simulink model "CML_Dyanmic_Sensory_Weighting"  (R2015a)
settings: Solver=ode4  SolverMode=MultiTasking  StartTime=0.0  StopTime=inf  FixedStep=BKIN_STEP_TIME  RelTol=1e-3
StartFcn:
  |  warndlg('Dexterit-E models cannot run under simulation. Please compile your model and run it from within Dexterit-E.');set_param(bdroot,'SimulationCommand','stop')
model workspace (MAT data in the model file):
  col_x = 1
  col_y = 2
  RADIUS_VIS = 3
  COLOR_INIT = 4
  START_TARGET_COL = 1
  DELAY_POST_TRIAL_COL = 17
  BKIN_STEP_TIME = 0.00025
  COLOR_MOVE = 5
  START_WAIT_TIME_COL = 2
  STIM_DUR_COL = 13
  MAX_MOVE_TIME_COL = 14
  HOLD_TIME_COL = 15
  E_START_TRIAL = 2
  E_START_REACHED = 4
  E_MOVED_EARLY = 21
  E_GO_CUE = 9
  E_MOVE_TIMEOUT = 23
  E_HOLDING_STILL = 12
  E_END_TRIAL = 14
  CONTROL_PT3_COL = 10
  STROKE_WIDTH = 6
  K_HAND_VEL = 1
  E_MOVE_ON = 10
  CUE_TYPE_COL = 6
  HAND_VIS_COL = 5
  K_HOLDTIME = 2
  K_ROBOT_RAMP_TIME = 3
  E_ROBOT_RETURN_TO_START = 33
  E_ENABLED_CONTROLLER = 31
  K_TIME_TO_START = 4
  E_RETURN_TO_START = 35
  E_HOLD_POS = 37
  E_INCREMENTING_TSTEP1 = 6
  E_INCREMENTING_TSTEP2 = 7
  E_INCREMENTING_TSTEP3 = 8
  CONTROL_PT0_COL = 7
  BKIN_KINEMATIC_FRAME_SIZE = 400
  E_NO_EVENT = 0
  E_BUTTON_ON = 40
  CONTROL_PTV1_COL = 8
  CONTROL_PTV2_COL = 9
  CONTROL_PTP1_COL = 11
  CONTROL_PTP2_COL = 12
  REACH_TARGET_COL = 3
  VIS_TARGET_COL = 4
  RADIUS_LOGICAL = 7
  FEEDBACK_TIME_COL = 16
  K_HAND_TARGET = 5
  E_SHOW_FEEDBACK = 16
  K_MIDPOINTY = 6
  K_MIDPOINT_Y = 6
  K_ARC_FDBK_TARGET = 7
  TEXT1 = 8
  TEXT2 = 9
  TEXT3 = 10
  K_CUE_TARGET = 8
  CONTINUE = 4
  TEXT4 = 11
  E_PAUSE = 41
libraries: slrtlib x10, Video x9, General x3, KINARM_general x3, KINARM_loads x2, xpcnilib x1
(part 1 of 2)
CloseFcn:
  | rtwprivate ssgencode ModelCloseRequest b2lab2d
settings Model: xpc_rtwmakecfg_data=_xpcethercatlib_  ModifiedComment=chris -- Wed Feb 16 09:18:30 2005 -- Version 1.1384  ModifiedHistory=Feb 16/05 - Add error repeat, add offset ramp  ExtModeArmWhenConnect=off  ExtModeLogAll=off  Creator=Chris Grebeldinger  LastModifiedBy=User
settings SolverCC: EnableConcurrentExecution=on  AutoInsertRateTranBlk=on
settings DataIOCC: LimitDataPoints=off  SignalLoggingSaveFormat=ModelDataLogs  SaveOutput=off  SaveTime=off  SignalLoggingName=sigsOut
settings OptimizationCC: BlockReduction=off  BooleanDataType=off  OptimizeBlockIOStorage=off  BufferReuse=off  GlobalBufferReuse=off  ExpressionFolding=off  ExpressionDepthLimit=2147483647  LocalBlockOutputs=off  InitFltsAndDblsToZero=on
settings DebuggingCC: SaveWithParameterizedLinksMsg=none  UnderspecifiedInitializationDetection=Classic  MergeDetectMultiDrivingBlocksExec=none  SignalResolutionControl=TryResolveAllWithWarning  MultiTaskDSMMsg=warning  FcnCallInpInsideContextMsg=UseLocalSettings  StateNameClashWarn=warning  StrictBusMsg=ErrorOnBusTreatedAsVector
settings HardwareCC: ProdIntDivRoundTo=Zero  ProdEndianess=LittleEndian  ProdLongLongMode=on  ProdHWDeviceType=Generic->32-bit x86 compatible  TargetHWDeviceType=32-bit Generic
settings SFSimCC: SimCustomHeaderCode="#include \"stdlib.h\""  SFSimEcho=off  SimParseCustomCode=off
settings RTWCC: SystemTargetFile=slrt.tlc  TemplateMakefile=slrt_default_tmf  Description=Simulink Real-Time  CustomSourceCode="#include \"stdlib.h\""
settings CodeAppCC: MaxIdLength=63
settings SimulinkRealTimeCC: TargetFcnLib=ansi_tfl_tmw.mat  GeneratePreprocessorConditionals=Disable all  xPCisDownloadable=off  xPCisDefaultEnv=off

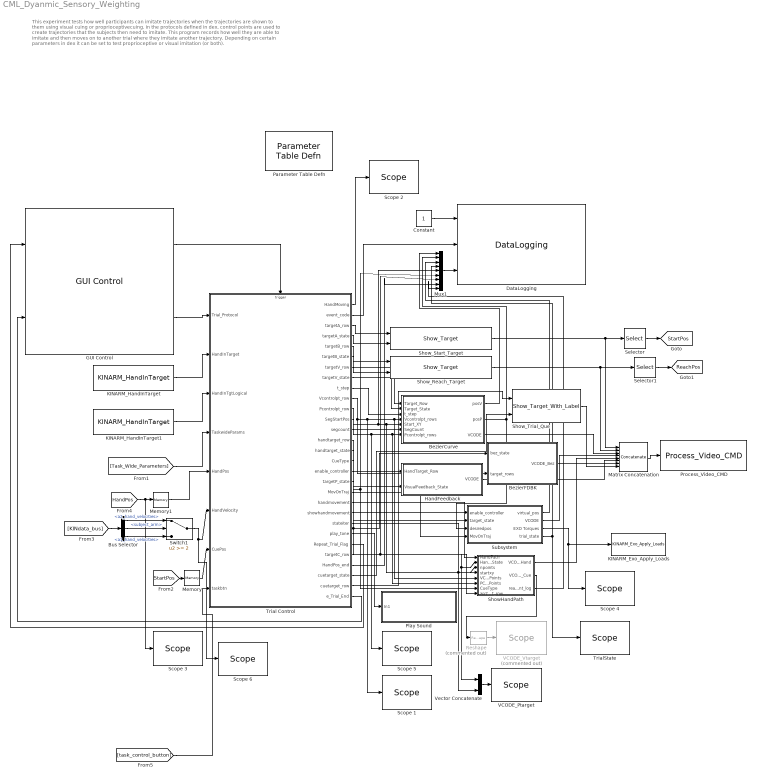
== system CML_Dyanmic_Sensory_Weighting ==
  note: This experiment tests how well participants can imitate trajectories when the trajectories
      | are shown to them using visual cuing or proprioceptivecuing. In the protocols defined in
      | dex, control points are used to create trajectories that the subjects then need to imitate.
      | This program records how well they are able to imitate and then moves on to another trial
      | where they imitate another trajectory. Depending on certain parameters in dex it can be
      | set to test proprioceptive or visual imitation (or both).
  BezierCurve : Subsystem
  BezierFDBK : Subsystem
  Bus Selector : BusSelector  OutputSignals=Robot2.a2_hand_velocities,KINDataGeneral.subject_arm,Robot1.a1_hand_velocities
  Constant : Constant
  DataLogging : General/DataLogging  log_event_codes=on  log_analog_inputs=on  show_time_remaining=off  ecat_include=on
  GUI Control : General/GUI Control  task_version=1.0  show_repeat_trial_flag=on  use_custom_tp=off  target_type_str=Circle  Target_Type=1  XYcols=[1 2]  Vcols=3  Lcols=4  indices_padding=[0 0 0 0;0 0 0 0]  target_table_rows=64  load_table_rows=20  tp_table_rows=100
  HandFeedback : Subsystem
  KINARM_Exo_Apply_Loads : KINARM_loads/KINARM_Exo_Apply_Loads  up_duration=200  down_duration=200  max_torque=5  limit_motors=off
  KINARM_HandInTarget : KINARM_general/KINARM_HandInTarget  use_dominant_hand=on  target_type=Circle  num_states=1  attribcol1=[RADIUS_VIS]  attribcol2=[0]  attribcol3=[0]  attribcol4=[0]  attribcol5=[0]
  KINARM_HandInTarget1 : KINARM_general/KINARM_HandInTarget  use_dominant_hand=on  target_type=Circle  num_states=1  attribcol1=[RADIUS_LOGICAL]  attribcol2=[0]  attribcol3=[0]  attribcol4=[0]  attribcol5=[0]
  Matrix Concatenation : Concatenate  NumInputs=8  Mode=Multidimensional array
  Memory : Memory
  Memory1 : Memory
  Mux1 : Mux  Inputs=9
  Parameter Table Defn : General/Parameter Table Defn  ShowInLibBrowser=0
  Play Sound : Subsystem
  Process_Video_CMD : Video/Process_Video_CMD  video_delay=50
  Reshape : Reshape  Commented=on
  Scope 1 : slrtlib/Displays and Logging/Scope   scopeno=7  scopetype=Target  autostart=on  viewmode=Numerical  formatstr='%15.6f'  grid=on  ylimits=[0,0]  nosamples=250  noprepostsamples=0  interleave=1  triggermode=FreeRun  triggersignal=1  trigsignalfromport=off  triggerlevel=0.0  triggerslope=Either  triggerscope=1  triggersample=0  filename=data.dat  mode=Lazy  writesize=512  autorestart=off  dynamicfilemode=off  maxwritefilesize=512*1024^2
  Scope 2 : slrtlib/Displays and Logging/Scope   scopeno=2  scopetype=Target  autostart=on  viewmode=Numerical  formatstr='%15.6f'  grid=on  ylimits=[0,0]  nosamples=250  noprepostsamples=0  interleave=1  triggermode=FreeRun  triggersignal=1  trigsignalfromport=off  triggerlevel=0.0  triggerslope=Either  triggerscope=1  triggersample=0  filename=data.dat  mode=Lazy  writesize=512  autorestart=off  dynamicfilemode=off  maxwritefilesize=512*1024^2
  Scope 3 : slrtlib/Displays and Logging/Scope   scopeno=3  scopetype=Target  autostart=on  viewmode=Numerical  formatstr='%15.6f'  grid=on  ylimits=[0,0]  nosamples=250  noprepostsamples=0  interleave=1  triggermode=FreeRun  triggersignal=1  trigsignalfromport=off  triggerlevel=0.0  triggerslope=Either  triggerscope=1  triggersample=0  filename=data.dat  mode=Lazy  writesize=512  autorestart=off  dynamicfilemode=off  maxwritefilesize=512*1024^2
  Scope 4 : slrtlib/Displays and Logging/Scope   scopeno=6  scopetype=Target  autostart=on  viewmode=Numerical  formatstr='%15.6f'  grid=on  ylimits=[0,0]  nosamples=250  noprepostsamples=0  interleave=1  triggermode=FreeRun  triggersignal=1  trigsignalfromport=off  triggerlevel=0.0  triggerslope=Either  triggerscope=1  triggersample=0  filename=data.dat  mode=Lazy  writesize=512  autorestart=off  dynamicfilemode=off  maxwritefilesize=512*1024^2
  Scope 5 : slrtlib/Displays and Logging/Scope   scopeno=8  scopetype=Target  autostart=on  viewmode=Numerical  formatstr='%15.6f'  grid=on  ylimits=[0,0]  nosamples=250  noprepostsamples=0  interleave=1  triggermode=FreeRun  triggersignal=1  trigsignalfromport=off  triggerlevel=0.0  triggerslope=Either  triggerscope=1  triggersample=0  filename=data.dat  mode=Lazy  writesize=512  autorestart=off  dynamicfilemode=off  maxwritefilesize=512*1024^2
  Scope 6 : slrtlib/Displays and Logging/Scope   scopeno=4  scopetype=Target  autostart=on  viewmode=Numerical  formatstr='%15.6f'  grid=on  ylimits=[0,0]  nosamples=250  noprepostsamples=0  interleave=1  triggermode=FreeRun  triggersignal=1  trigsignalfromport=off  triggerlevel=0.0  triggerslope=Either  triggerscope=1  triggersample=0  filename=data.dat  mode=Lazy  writesize=512  autorestart=off  dynamicfilemode=off  maxwritefilesize=512*1024^2
  Selector : Selector  InputPortWidth=70  Indices=[3 4]
  Selector1 : Selector  InputPortWidth=70  Indices=[3 4]
  ShowHandPath : Subsystem
  Show_Reach_Target : Video/Show_Target  target_type=Rectangle  num_states=1  attribcol1=[0 COLOR_INIT STROKE_WIDTH RADIUS_VIS RADIUS_VIS 0]  attribcol2=[0 0 0 0 0 0]  attribcol3=[0 0 0 0 0 0]  attribcol4=[0 0 0 0 0 0]  attribcol5=[0 0 0 0 0 0]  stateindices_padding=[0 0 0 0 0;0 0 0 0 0;0 0 0 0 0;0 0 0 0 0;0 0 0 0 0]  source=dialog  opacity=100  target_display=Both subject and operator displays  num_col=6
  Show_Start_Target : Video/Show_Target  target_type=Rectangle  num_states=1  attribcol1=[0 COLOR_INIT STROKE_WIDTH RADIUS_VIS RADIUS_VIS 0]  attribcol2=[0 0 0 0 0 0]  attribcol3=[0 0 0 0 0 0]  attribcol4=[0 0 0 0 0 0]  attribcol5=[0 0 0 0 0 0]  stateindices_padding=[0 0 0 0 0;0 0 0 0 0;0 0 0 0 0;0 0 0 0 0;0 0 0 0 0]  source=dialog  opacity=100  target_display=Both subject and operator displays  num_col=6
  Show_Trial_Que : Video/Show_Target_With_Label  target_type=Circle  num_states=4  attribcol1=[0 0 0 RADIUS_VIS TEXT1 COLOR_INIT STROKE_WIDTH]  attribcol2=[0 0 0 RADIUS_VIS TEXT2 COLOR_INIT STROKE_WIDTH]  attribcol3=[0 0 0 RADIUS_VIS TEXT3 COLOR_INIT STROKE_WIDTH]  attribcol4=[0 0 0 RADIUS_VIS TEXT4 COLOR_INIT STROKE_WIDTH]  attribcol5=[0 0 0 0 0 0 0]  stateindices_padding=[0 0 0 0;0 0 0 0;0 0 0 0;0 0 0 0;0 0 0 0]  source=dialog  opacity=100  target_display=Both subject and operator displays
  Subsystem : Subsystem
  Switch1 : Switch  Threshold=2
  Trial Control : Stateflow chart  TreatAsAtomicUnit=on
  TrialState : slrtlib/Displays and Logging/Scope   scopeno=1  scopetype=Target  autostart=on  viewmode=Numerical  formatstr='%15.6f'  grid=on  ylimits=[0,0]  nosamples=250  noprepostsamples=0  interleave=1  triggermode=FreeRun  triggersignal=1  trigsignalfromport=off  triggerlevel=0.0  triggerslope=Either  triggerscope=1  triggersample=0  filename=data.dat  mode=Lazy  writesize=512  autorestart=off  dynamicfilemode=off  maxwritefilesize=512*1024^2
  VCODE_Ptarget : slrtlib/Displays and Logging/Scope   scopeno=5  scopetype=Target  autostart=on  viewmode=Numerical  formatstr='%15.6f'  grid=on  ylimits=[0,0]  nosamples=250  noprepostsamples=0  interleave=1  triggermode=FreeRun  triggersignal=1  trigsignalfromport=off  triggerlevel=0.0  triggerslope=Either  triggerscope=1  triggersample=0  filename=data.dat  mode=Lazy  writesize=512  autorestart=off  dynamicfilemode=off  maxwritefilesize=512*1024^2
  VCODE_Vtarget : slrtlib/Displays and Logging/Scope   Commented=on  scopeno=4  scopetype=Target  autostart=on  viewmode=Numerical  formatstr='%15.6f'  grid=on  ylimits=[0,0]  nosamples=250  noprepostsamples=0  interleave=1  triggermode=FreeRun  triggersignal=1  trigsignalfromport=off  triggerlevel=0.0  triggerslope=Either  triggerscope=1  triggersample=0  filename=data.dat  mode=Lazy  writesize=512  autorestart=off  dynamicfilemode=off  maxwritefilesize=512*1024^2
  Vector Concatenate : Concatenate
  tag scope: ReachPos=global, StartPos=global
  wires:
  Trial Control/29(e_Trial_End) -> GUI Control/2
  Trial Control/4(targetA_state) -> Show_Start_Target/2
  Trial Control/3(targetA_row) -> Show_Start_Target/1
  Matrix Concatenation/1 -> Process_Video_CMD/1
  Trial Control/2(event_code) -> DataLogging/2
  Constant/1 -> DataLogging/1
  GUI Control/2 -> Trial Control/1(Trial_Protocol)
  KINARM_HandInTarget/1 -> Trial Control/2(HandInTarget)
  Trial Control/14(handtarget_row) -> HandFeedback/1(HandTarget_Row)
  Trial Control/15(handtarget_state) -> HandFeedback/2(VisualFeedback_State)
  Show_Start_Target/1 -> Matrix Concatenation/1, Selector/1
  Trial Control/24(Repeat_Trial_Flag) -> GUI Control/1
  [Task_Wide_Parameters] -> Trial Control/4(TaskwideParams)
  Trial Control/9(t_step) -> BezierCurve/3(t_step)
  Trial Control/7(targetV_row) -> BezierCurve/1(Target_Row)
  Trial Control/10(Vcontrolpt_row) -> BezierFDBK/2(target_rows), ShowHandPath/5(VControl_Points), BezierCurve/4(Vcontrolpt_rows), Scope 1/1
  Trial Control/1(HandMoving) -> Scope 2/1
  Switch1/1 -> Scope 6/1, Trial Control/6(HandVelocity)
  Trial Control/17(enable_controller) -> Subsystem/1(enable_controller)
  Trial Control/19(MovOnTraj) -> Subsystem/4(MovOnTraj)
  Mux1/1 -> DataLogging/3
  Subsystem/1(virtual_pos) -> Mux1/3
  Subsystem/3(EXO Torques) -> Scope 4/1, KINARM_Exo_Apply_Loads/1
  Subsystem/2(VCODE) -> Matrix Concatenation/4
  BezierCurve/3(VCODE) -> Matrix Concatenation/3
  Subsystem/4(trial_state) -> TrialState/1, Mux1/4
  [KINdata_bus] -> Bus Selector/1
  Trial Control/8(targetV_state) -> BezierCurve/2(Target_State)
  Trial Control/12(SegStartPos) -> Mux1/5, ShowHandPath/4(startxy), BezierCurve/5(Start_XY)
  HandFeedback/1(VCODE) -> Matrix Concatenation/6
  BezierCurve/1(posV) -> Mux1/1
  Memory/1 -> Trial Control/7(CuePos)
  Trial Control/13(segcount) -> BezierCurve/6(SegCount)
  Trial Control/23(play_tone) -> Play Sound/1(In1)
  GUI Control/1 -> Trial Control/Trigger
  BezierCurve/2(posP) -> Mux1/2, Subsystem/3(desiredpos)
  Trial Control/18(targetP_state) -> Subsystem/2(target_state)
  Trial Control/11(Pcontrolpt_row) -> Scope 5/1, ShowHandPath/6(PControl_Points), BezierCurve/7(Pcontrolpt_rows)
  Selector/1 -> [StartPos]
  [StartPos] -> Memory/1
  Trial Control/5(targetB_row) -> Show_Reach_Target/1
  Trial Control/6(targetB_state) -> Show_Reach_Target/2
  KINARM_HandInTarget1/1 -> Trial Control/3(HandInTgtLogical)
  Trial Control/16(CueType) -> ShowHandPath/7(CueType), Mux1/6
  [HandPos] -> Scope 3/1, Memory1/1
  Memory1/1 -> Trial Control/5(HandPos)
  Trial Control/20(handmovement) -> ShowHandPath/1(HandPath)
  Trial Control/21(showhandmovement) -> BezierFDBK/1("bez_state "), Vector Concatenate/1, ShowHandPath/2(HandPathState), Mux1/7
  ShowHandPath/1(VCODE_Hand) -> Matrix Concatenation/5
  Trial Control/22(stateiter) -> Vector Concatenate/2, ShowHandPath/3(npoints)
  Vector Concatenate/1 -> VCODE_Ptarget/1
  Reshape/1 -> VCODE_Vtarget/1
  ShowHandPath/3("reachmidpoint_log ") -> Mux1/9
  Trial Control/25(targetC_row) -> ShowHandPath/8(arctarget_row)
  Show_Reach_Target/1 -> Selector1/1, Matrix Concatenation/2
  Selector1/1 -> [ReachPos]
  BezierFDBK/1(VCODE_Bez) -> Matrix Concatenation/7
  Bus Selector/3 -> Switch1/3  "<a1_hand_velocities>"
  Bus Selector/2 -> Switch1/2  "<subject_arm>"
  Bus Selector/1 -> Switch1/1  "<a2_hand_velocities>"
  Trial Control/26(HandPos_end) -> Mux1/8
  ShowHandPath/2(VCODE_Cue) -> Reshape/1
  Show_Trial_Que/1 -> Matrix Concatenation/8
  Trial Control/27(cuetarget_state) -> Show_Trial_Que/2
  Trial Control/28(cuetarget_row) -> Show_Trial_Que/1
  [task_control_button] -> Trial Control/8(taskbtn)

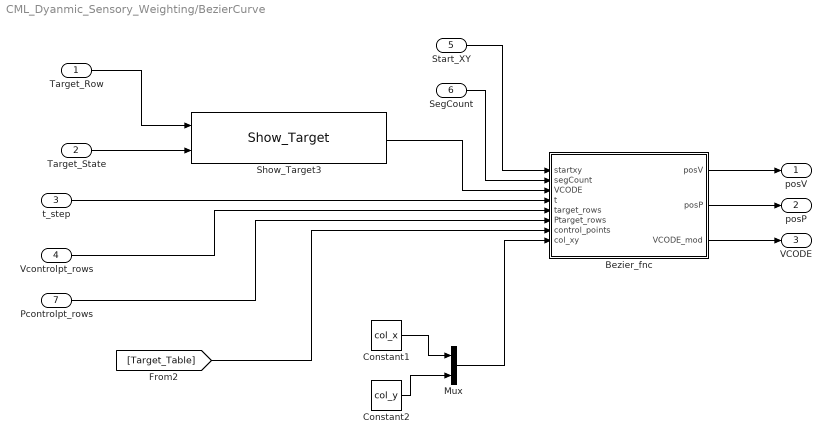
== system CML_Dyanmic_Sensory_Weighting/BezierCurve ==
  Target_Row : Inport
  Target_State : Inport  Port=2
  t_step : Inport  Port=3
  Vcontrolpt_rows : Inport  Port=4
  Start_XY : Inport  Port=5
  SegCount : Inport  Port=6
  Pcontrolpt_rows : Inport  Port=7
  Bezier_fnc : MATLAB Function  TreatAsAtomicUnit=on
  Constant1 : Constant  Value=col_x
  Constant2 : Constant  Value=col_y
  Mux : Mux  Inputs=2
  Show_Target3 : Video/Show_Target  target_type=Circle  num_states=1  attribcol1=[COLOR_INIT 0 0 RADIUS_VIS]  attribcol2=[0 0 0 0]  attribcol3=[0 0 0 0]  attribcol4=[0 0 0 0]  attribcol5=[0 0 0 0]  stateindices_padding=[0 0 0 0 0 0 0;0 0 0 0 0 0 0;0 0 0 0 0 0 0;0 0 0 0 0 0 0;0 0 0 0 0 0 0]  source=dialog  opacity=100  target_display=Both subject and operator displays  num_col=4
  posV : Outport
  posP : Outport  Port=2
  VCODE : Outport  Port=3
  wires:
  Show_Target3/1 -> Bezier_fnc/3(VCODE)
  Bezier_fnc/3(VCODE_mod) -> VCODE/1
  t_step/1 -> Bezier_fnc/4(t)
  [Target_Table] -> Bezier_fnc/7(control_points)
  Vcontrolpt_rows/1 -> Bezier_fnc/5(target_rows)
  Bezier_fnc/1(posV) -> posV/1
  Target_Row/1 -> Show_Target3/1
  Target_State/1 -> Show_Target3/2
  Mux/1 -> Bezier_fnc/8(col_xy)
  Constant1/1 -> Mux/1
  Constant2/1 -> Mux/2
  Start_XY/1 -> Bezier_fnc/1(startxy)
  SegCount/1 -> Bezier_fnc/2(segCount)
  Bezier_fnc/2(posP) -> posP/1
  Pcontrolpt_rows/1 -> Bezier_fnc/6(Ptarget_rows)

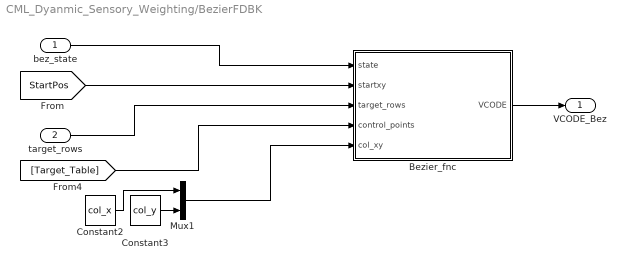
== system CML_Dyanmic_Sensory_Weighting/BezierFDBK ==
  "bez_state " : Inport
  target_rows : Inport  Port=2
  Bezier_fnc : MATLAB Function  TreatAsAtomicUnit=on
  Constant2 : Constant  Value=col_x
  Constant3 : Constant  Value=col_y
  Mux1 : Mux  Inputs=2
  VCODE_Bez : Outport
  wires:
  [Target_Table] -> Bezier_fnc/4(control_points)
  "bez_state "/1 -> Bezier_fnc/1(state)
  Constant2/1 -> Mux1/1
  Constant3/1 -> Mux1/2
  Mux1/1 -> Bezier_fnc/5(col_xy)
  target_rows/1 -> Bezier_fnc/3(target_rows)
  Bezier_fnc/1(VCODE) -> VCODE_Bez/1
  [StartPos] -> Bezier_fnc/2(startxy)

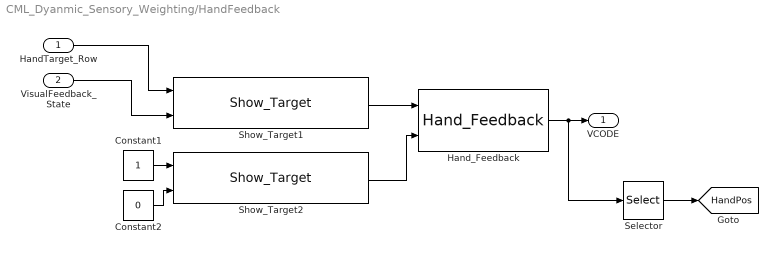
== system CML_Dyanmic_Sensory_Weighting/HandFeedback ==
  HandTarget_Row : Inport
  VisualFeedback_State : Inport  Port=2
  Constant1 : Constant
  Constant2 : Constant  Value=0
  Hand_Feedback : KINARM_general/Hand_Feedback  feedback_cntl_src=style and status
  Selector : Selector  NumberOfDimensions=2  InputPortWidth=70  IndexOptions=Index vector (dialog),Index vector (dialog)  Indices=1,[3 4]  OutputSizes=1,1
  Show_Target1 : Video/Show_Target  target_type=Circle  num_states=2  attribcol1=[COLOR_INIT 0 0 RADIUS_VIS]  attribcol2=[COLOR_MOVE 0 0 RADIUS_VIS]  attribcol3=[0 0 0 0]  attribcol4=[0 0 0 0]  attribcol5=[0 0 0 0]  stateindices_padding=[0 0 0 0 0 0 0;0 0 0 0 0 0 0;0 0 0 0 0 0 0;0 0 0 0 0 0 0;0 0 0 0 0 0 0]  source=dialog  opacity=100  target_display=Both subject and operator displays  num_col=4
  Show_Target2 : Video/Show_Target  target_type=Circle  num_states=2  attribcol1=[COLOR_INIT 0 0 RADIUS_VIS]  attribcol2=[COLOR_MOVE 0 0 RADIUS_VIS]  attribcol3=[0 0 0 0]  attribcol4=[0 0 0 0]  attribcol5=[0 0 0 0]  stateindices_padding=[0 0 0 0 0 0 0;0 0 0 0 0 0 0;0 0 0 0 0 0 0;0 0 0 0 0 0 0;0 0 0 0 0 0 0]  source=dialog  opacity=100  target_display=Both subject and operator displays  num_col=4
  VCODE : Outport
  tag scope: HandPos=global
  wires:
  Show_Target1/1 -> Hand_Feedback/1
  HandTarget_Row/1 -> Show_Target1/1
  VisualFeedback_State/1 -> Show_Target1/2
  Constant1/1 -> Show_Target2/1
  Constant2/1 -> Show_Target2/2
  Show_Target2/1 -> Hand_Feedback/2
  Hand_Feedback/1 -> Selector/1, VCODE/1
  Selector/1 -> [HandPos]

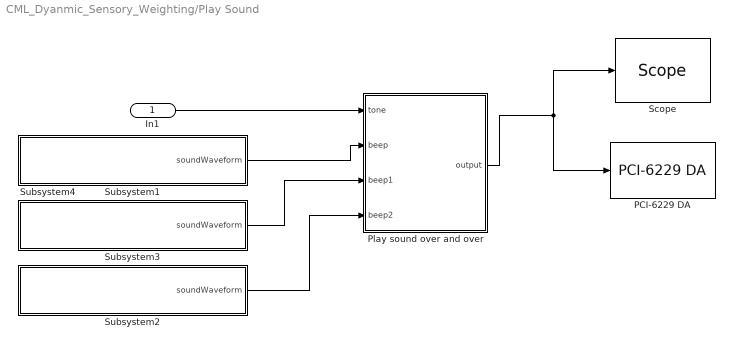
== system CML_Dyanmic_Sensory_Weighting/Play Sound ==
  In1 : Inport
  PCI-6229 DA : xpcnilib/D//A/M Series/PCI-6229 DA  channel=[1]  reset=[1]  initValue=[0]  sampletime=-1  slot=-1
  Play sound over and over : MATLAB Function  TreatAsAtomicUnit=on
  "Scope " : slrtlib/Displays and Logging/Scope   scopeno=9  scopetype=Target  autostart=on  viewmode=Graphical redraw  formatstr='%15.6f'  grid=on  ylimits=[0,0]  nosamples=4000  noprepostsamples=0  interleave=1  triggermode=FreeRun  triggersignal=1  trigsignalfromport=off  triggerlevel=0.0  triggerslope=Either  triggerscope=1  triggersample=0  filename=data.dat  mode=Lazy  writesize=512  autorestart=off  dynamicfilemode=off  maxwritefilesize=512*1024^2
  Subsystem1 : Subsystem  mask(Load Waveform Into Variable){fileName=beep}
      mask prompts: fileName "Name of .mat Data File (must be in current directory)"
      mask help: This block will load the .MAT file specified in the dialog, and put the first variable into a GoTo called 'soundWaveform'.
      mask init:
      | filenameFromMask = get_param(gcb, 'fileName');
      | 
      | try 
      | 	dataFromFile = load(filenameFromMask);
      | 	names = fieldnames(dataFromFile);
      | 	soundDataFromFile = dataFromFile.(names{1});
      | 	display(['Sound waveform from file ''' filenameFromMask ''' loaded.']);
      | catch ME
      | 	display(ME.message)
      | end
      mask Help:
      | Enter the name a .MAT file containing a single vector or matrix. The .MAT file must be located in the current directory.
      | 
      | The first variable from the .MAT file will be put into a Goto called 'soundWaveform'.
      mask Display: disp(['Load waveform from ''' filenameFromMask ''''])
  Subsystem2 : Subsystem  mask(Load Waveform Into Variable){fileName=beep2}
      mask prompts: fileName "Name of .mat Data File (must be in current directory)"
      mask help: This block will load the .MAT file specified in the dialog, and put the first variable into a GoTo called 'soundWaveform'.
      mask init: same as CML_Dyanmic_Sensory_Weighting/Play Sound/Subsystem1
      mask Help:
      | Enter the name a .MAT file containing a single vector or matrix. The .MAT file must be located in the current directory.
      | 
      | The first variable from the .MAT file will be put into a Goto called 'soundWaveform'.
      mask Display: disp(['Load waveform from ''' filenameFromMask ''''])
  Subsystem3 : Subsystem  mask(Load Waveform Into Variable){fileName=beep1}
      mask prompts: fileName "Name of .mat Data File (must be in current directory)"
      mask help: This block will load the .MAT file specified in the dialog, and put the first variable into a GoTo called 'soundWaveform'.
      mask init: same as CML_Dyanmic_Sensory_Weighting/Play Sound/Subsystem1
      mask Help:
      | Enter the name a .MAT file containing a single vector or matrix. The .MAT file must be located in the current directory.
      | 
      | The first variable from the .MAT file will be put into a Goto called 'soundWaveform'.
      mask Display: disp(['Load waveform from ''' filenameFromMask ''''])
  Subsystem4 : Subsystem  mask(Load Waveform Into Variable){fileName=beep}
      mask prompts: fileName "Name of .mat Data File (must be in current directory)"
      mask help: This block will load the .MAT file specified in the dialog, and put the first variable into a GoTo called 'soundWaveform'.
      mask init: same as CML_Dyanmic_Sensory_Weighting/Play Sound/Subsystem1
      mask Help:
      | Enter the name a .MAT file containing a single vector or matrix. The .MAT file must be located in the current directory.
      | 
      | The first variable from the .MAT file will be put into a Goto called 'soundWaveform'.
      mask Display: disp(['Load waveform from ''' filenameFromMask ''''])
  wires:
  Play sound over and over/1(output) -> PCI-6229 DA/1, "Scope "/1
  Subsystem3/1(soundWaveform) -> Play sound over and over/3(beep1)
  Subsystem4/1(soundWaveform) -> Play sound over and over/2(beep)
  In1/1 -> Play sound over and over/1(tone)
  Subsystem2/1(soundWaveform) -> Play sound over and over/4(beep2)

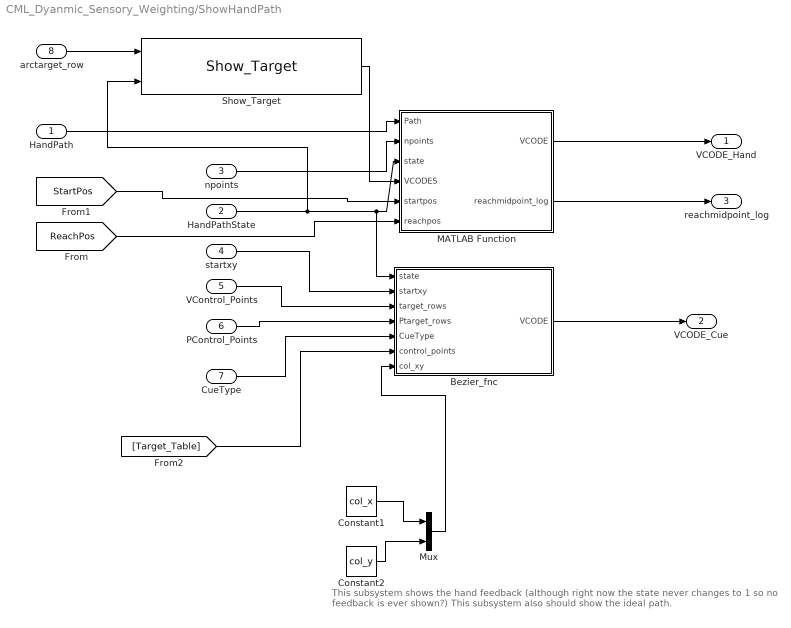
== system CML_Dyanmic_Sensory_Weighting/ShowHandPath ==
  note: This subsystem shows the hand feedback (although right now the state never changes to 1 so no feedback is ever shown?)
      |
      | This subsystem also should show the ideal path.
  HandPath : Inport
  HandPathState : Inport  Port=2
  npoints : Inport  Port=3
  startxy : Inport  Port=4
  VControl_Points : Inport  Port=5
  PControl_Points : Inport  Port=6
  CueType : Inport  Port=7
  arctarget_row : Inport  Port=8
  Bezier_fnc : MATLAB Function  TreatAsAtomicUnit=on
  Constant1 : Constant  Value=col_x
  Constant2 : Constant  Value=col_y
  MATLAB Function : MATLAB Function  TreatAsAtomicUnit=on
  Mux : Mux  Inputs=2
  Show_Target : Video/Show_Target  target_type=Circle  num_states=1  attribcol1=[COLOR_INIT 0 0 RADIUS_VIS]  attribcol2=[0 0 0 0]  attribcol3=[0 0 0 0]  attribcol4=[0 0 0 0]  attribcol5=[0 0 0 0]  stateindices_padding=[0 0 0 0 0 0 0;0 0 0 0 0 0 0;0 0 0 0 0 0 0;0 0 0 0 0 0 0;0 0 0 0 0 0 0]  source=dialog  opacity=100  target_display=Both subject and operator displays  num_col=4
  VCODE_Hand : Outport
  VCODE_Cue : Outport  Port=2
  "reachmidpoint_log " : Outport  Port=3
  wires:
  MATLAB Function/1(VCODE) -> VCODE_Hand/1
  MATLAB Function/2(reachmidpoint_log) -> "reachmidpoint_log "/1
  npoints/1 -> MATLAB Function/2(npoints)
  HandPathState/1 -> Show_Target/2, Bezier_fnc/1(state), MATLAB Function/3(state)
  startxy/1 -> Bezier_fnc/2(startxy)
  VControl_Points/1 -> Bezier_fnc/3(target_rows)
  PControl_Points/1 -> Bezier_fnc/4(Ptarget_rows)
  [Target_Table] -> Bezier_fnc/6(control_points)
  Mux/1 -> Bezier_fnc/7(col_xy)
  Constant1/1 -> Mux/1
  Constant2/1 -> Mux/2
  CueType/1 -> Bezier_fnc/5(CueType)
  Bezier_fnc/1(VCODE) -> VCODE_Cue/1
  HandPath/1 -> MATLAB Function/1(Path)
  arctarget_row/1 -> Show_Target/1
  Show_Target/1 -> MATLAB Function/4(VCODES)
  [StartPos] -> MATLAB Function/5(startpos)
  [ReachPos] -> MATLAB Function/6(reachpos)

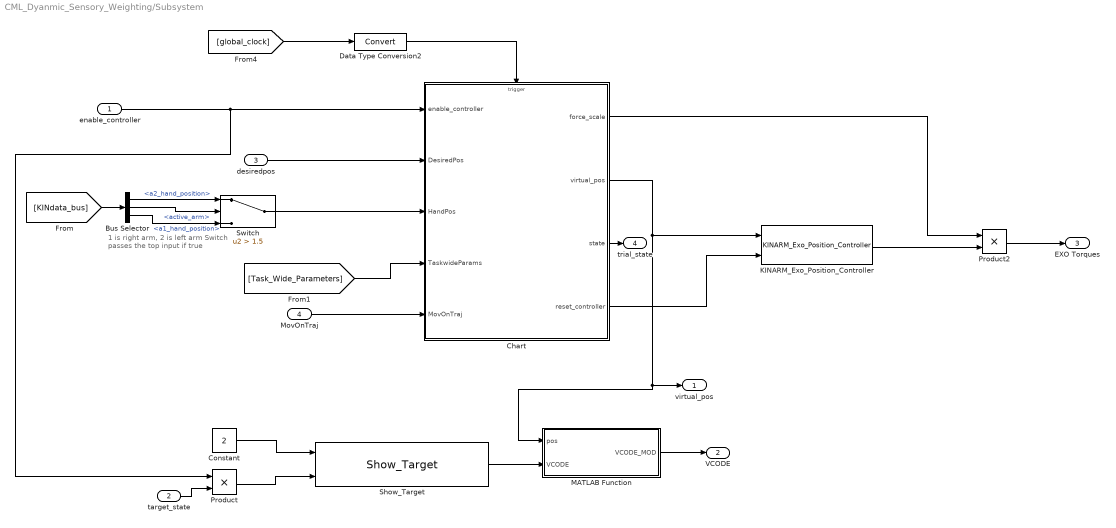
== system CML_Dyanmic_Sensory_Weighting/Subsystem ==
  note: 1 is right arm, 2 is left arm
      | Switch passes the top input if true
  enable_controller : Inport
  target_state : Inport  Port=2
  desiredpos : Inport  Port=3
  MovOnTraj : Inport  Port=4
  Bus Selector : BusSelector  OutputSignals=Robot2.a2_hand_position,KINDataGeneral.active_arm,Robot1.a1_hand_position
  Chart : Stateflow chart  TreatAsAtomicUnit=on
  Constant : Constant  Value=2
  Data Type Conversion2 : DataTypeConversion
  KINARM_Exo_Position_Controller : KINARM_loads/KINARM_Exo_Position_Controller  use_dom_hand=on  KINARM_Type=Human  inertias_for_FF=KINARM robot & arm troughs & subject  angles_or_XY=End-point (global x/y)  sample_time=0.001
  MATLAB Function : MATLAB Function  TreatAsAtomicUnit=on
  Product : Product
  Product2 : Product
  Show_Target : Video/Show_Target  target_type=Circle  num_states=1  attribcol1=[COLOR_INIT 0 0 RADIUS_VIS]  attribcol2=[0 0 0 0]  attribcol3=[0 0 0 0]  attribcol4=[0 0 0 0]  attribcol5=[0 0 0 0]  stateindices_padding=[0 0 0 0 0 0 0;0 0 0 0 0 0 0;0 0 0 0 0 0 0;0 0 0 0 0 0 0;0 0 0 0 0 0 0]  source=dialog  opacity=100  target_display=Both subject and operator displays  num_col=4
  Switch : Switch  Criteria=u2 > Threshold  Threshold=1.5
  virtual_pos : Outport
  VCODE : Outport  Port=2
  EXO Torques : Outport  Port=3
  trial_state : Outport  Port=4
  wires:
  [KINdata_bus] -> Bus Selector/1
  Bus Selector/2 -> Switch/2  "<active_arm>"
  [Task_Wide_Parameters] -> Chart/4(TaskwideParams)
  [global_clock] -> Data Type Conversion2/1
  Data Type Conversion2/1 -> Chart/Trigger
  Chart/2(virtual_pos) -> MATLAB Function/1(pos), virtual_pos/1, KINARM_Exo_Position_Controller/1
  MovOnTraj/1 -> Chart/5(MovOnTraj)
  Switch/1 -> Chart/3(HandPos)
  desiredpos/1 -> Chart/2(DesiredPos)
  Constant/1 -> Show_Target/1
  Show_Target/1 -> MATLAB Function/2(VCODE)
  MATLAB Function/1(VCODE_MOD) -> VCODE/1
  KINARM_Exo_Position_Controller/1 -> Product2/2
  Product2/1 -> EXO Torques/1
  Chart/1(force_scale) -> Product2/1
  Chart/4(reset_controller) -> KINARM_Exo_Position_Controller/2
  Bus Selector/1 -> Switch/1  "<a2_hand_position>"
  Bus Selector/3 -> Switch/3  "<a1_hand_position>"
  Chart/3(state) -> trial_state/1
  enable_controller/1 -> Product/1, Chart/1(enable_controller)
  Product/1 -> Show_Target/2
  target_state/1 -> Product/2

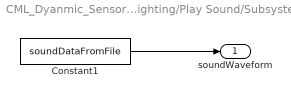
== system CML_Dyanmic_Sensory_Weighting/Play Sound/Subsystem1 ==
  Constant1 : Constant  Value=soundDataFromFile
  soundWaveform : Outport
  wires:
  Constant1/1 -> soundWaveform/1

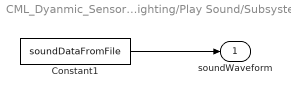
== system CML_Dyanmic_Sensory_Weighting/Play Sound/Subsystem2 ==
  Constant1 : Constant  Value=soundDataFromFile
  soundWaveform : Outport
  wires:
  Constant1/1 -> soundWaveform/1

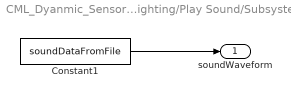
== system CML_Dyanmic_Sensory_Weighting/Play Sound/Subsystem3 ==
  Constant1 : Constant  Value=soundDataFromFile
  soundWaveform : Outport
  wires:
  Constant1/1 -> soundWaveform/1

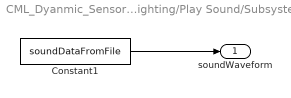
== system CML_Dyanmic_Sensory_Weighting/Play Sound/Subsystem4 ==
  Constant1 : Constant  Value=soundDataFromFile
  soundWaveform : Outport
  wires:
  Constant1/1 -> soundWaveform/1

== stateflow chart CML_Dyanmic_Sensory_Weighting/Subsystem/Chart ==
  state EnableState/
    state AutoMoveToPos/
      //smoothly creates a trajectory to get the hand to a point eventually
      state MovingToDesiredXY/
        tickCount = TaskwideParams[K_TIME_TO_START];
        state = 11;
        tick = 0;
        during:
        on e_clk: tick++;
        // the trajectory velocity will have a bell shaped profile
        trajectory_shape = tick/tickCount-sin(2*pi*tick/tickCount)/(2*pi);
        virtual_pos[1] = StartPos[1] + (TgtPos[1] - StartPos[1]) * trajectory_shape;
        virtual_pos[2] = StartPos[2] + (TgtPos[2] - StartPos[2]) * trajectory_shape;
      state GetDesiredXY/
        //grab the current desired pos in case it changes
        TgtPos[1] = DesiredPos[1];
        TgtPos[2] = DesiredPos[2];
        StartPos[1] = HandPos[1];
        StartPos[2] = HandPos[2];
        updatepos = 0;
        state = 10;
      state HoldAtDesiredXY/
        //pause until something changes
        state = 12;
        updatepos = 0;
        during:
        on e_clk: updatepos = ( (abs(TgtPos[1]-DesiredPos[1]) > 0.01) || (abs(TgtPos[2]-DesiredPos[2]) > 0.01) )
      GetDesiredXY -> MovingToDesiredXY : after(1, e_clk)
      HoldAtDesiredXY -> GetDesiredXY : [updatepos == 1 && MovOnTraj == 0]
      MovingToDesiredXY -> HoldAtDesiredXY : after(tickCount, e_clk)/
    state MoveAlongTraj/
      //take a step along a trajectory specified externally
      state GetDesiredXY_Traj/
        TgtPos[1] = DesiredPos[1];
        TgtPos[2] = DesiredPos[2];
        StartPos[1] = HandPos[1];
        StartPos[2] = HandPos[2];
        state = 21;
        //movIsSafe = ( (abs(TgtPos[1]-HandPos[1]) < 0.02) || (abs(TgtPos[2]-HandPos[2]) < 0.02) );
        movIsSafe = 1;
      state MovAlongTraj/
        state = 22;
        virtual_pos[1] = DesiredPos[1];
        virtual_pos[2] = DesiredPos[2];
      GetDesiredXY_Traj -> MovAlongTraj [order 2] : [movIsSafe == 1]
      MovAlongTraj -> GetDesiredXY_Traj
    (junction 15) -> GetDesiredXY [order 1] : [MovOnTraj == 0]
    (junction 15) -> GetDesiredXY_Traj [order 2] : [MovOnTraj == 1]
    MoveAlongTraj -> GetDesiredXY : [MovOnTraj == 0]
    GetDesiredXY_Traj -> GetDesiredXY [order 1] : [movIsSafe == 0]
    AutoMoveToPos -> GetDesiredXY_Traj : [MovOnTraj == 1]
  state Init/
    ramp_time = TaskwideParams[K_ROBOT_RAMP_TIME];
    scale_increment = 1/ramp_time;
    force_scale = 0;
    state = 1;
    during:
    CurHandPos[1] = HandPos[1];
    CurHandPos[2] = HandPos[2];
  state RampUp/
    //ramp up the force scale to 1
    CurHandPos[1] = HandPos[1];
    CurHandPos[2] = HandPos[2];
    virtual_pos[1] = HandPos[1];
    virtual_pos[2] = HandPos[2];
    state = 2;
    force_scale = 0;
    during:
    on e_clk: force_scale += scale_increment;
  state ResetController/
    reset_controller;
  state RampDown/
    //ramp down the force scale to 1
    CurHandPos[1] = HandPos[1];
    CurHandPos[2] = HandPos[2];
    virtual_pos[1] = CurHandPos[1];
    virtual_pos[2] = CurHandPos[2];
    state = 30
    during:
    on e_clk: force_scale -= scale_increment;
  (default) -> Init
  Init -> ResetController : //if controller becomes enabled
      | [enable_controller == 1]/
      | force_scale = 0;
  ResetController -> RampUp
  RampUp -> (junction 15) [order 2] : [force_scale >= 1]/
      | force_scale = 1;
  RampDown -> Init [order 2] : [force_scale <0]/
      | force_scale = 0;
  RampDown -> RampUp [order 1] : [enable_controller == 1]
      | //if the controller is enabled
  RampUp -> RampDown [order 1] : [enable_controller == 0]
      | //if the controller gets shut off
  EnableState -> RampDown : [enable_controller == 0]
  data: enable_controller input boolean; DesiredPos input; HandPos input; TaskwideParams input; force_scale output double; virtual_pos output double size=2; tickCount local double; StartPos local double size=2; TgtPos local double size=2; updatepos local boolean; MovOnTraj input double; CurHandPos local double size=2; ramp_time local double; scale_increment local double; tick local double; trajectory_shape local double; movIsSafe local boolean; pi constant double =3.14159265358979; state output double
  events: e_clk input EITHER_EDGE_EVENT; reset_controller output EITHER_EDGE_EVENT

== stateflow chart CML_Dyanmic_Sensory_Weighting/Trial Control ==
  state MainTrial
    state InitPauseTrial/
      // Just want to pause for a little
      event_code = E_PAUSE;
    state ShowStartTarget/
      // Turn on start target
      event_code = E_START_TRIAL;
      targetA_row = Trial_Protocol[START_TARGET_COL];
      targetA_state = 1;
      targetB_row = Trial_Protocol[REACH_TARGET_COL];
      targetB_state = 0;
      targetC_row = TaskwideParams[K_ARC_FDBK_TARGET];
      targetV_row = Trial_Protocol[VIS_TARGET_COL];
      targetV_state = 0;
      enable_controller = 0;
      SegStartPos[1] = 0;
      SegStartPos[2] = 0;
      showhandmovement = 0;
      CueType = Trial_Protocol[CUE_TYPE_COL];
      cuetarget_row = TaskwideParams[K_CUE_TARGET];
    state RampOnController/
      SegStartPos[1] = 0.0;
      SegStartPos[2] = 0.0;
      segcount = 0;
      Vcontrolpt_row[1] = Trial_Protocol[START_TARGET_COL];
      Vcontrolpt_row[2] = -1;
      Vcontrolpt_row[3] = -1;
      Vcontrolpt_row[4] = -1;
      Pcontrolpt_row[1] = Trial_Protocol[START_TARGET_COL];
      Pcontrolpt_row[2] = -1;
      Pcontrolpt_row[3] = -1;
      Pcontrolpt_row[4] = -1;
      t_step = 0;
      event_code = E_ENABLED_CONTROLLER;
      MovOnTraj = 0;
      enable_controller = 1;
    state HoldAtStart/
      // Log an event that target was reached and then wait for a specified time.
      tickCount = Trial_Protocol[START_WAIT_TIME_COL] ;
      t_step = 0;
      %CueType = Trial_Protocol[CUE_TYPE_COL];
      targetV_row = Trial_Protocol[VIS_TARGET_COL];
      targetV_state = ((Trial_Protocol[CUE_TYPE_COL] == 0) || (Trial_Protocol[CUE_TYPE_COL] == 2)  || (Trial_Protocol[CUE_TYPE_COL] == 3)); //turn on for a V or VP target type
      //targetP_state = ((Trial_Protocol[CUE_TYPE_COL] == 1) || (Trial_Protocol[CUE_TYPE_COL] == 2)) && (Trial_Protocol[HAND_VIS_COL] == 1);
      targetP_state = 0; //we will use the hand feedback cursor instead
      handtarget_state = 1;
      t_step = 0;
      SegStartPos[1] = 0;
      SegStartPos[2] = 0;
      segcount = 0;
    state MoveToStart/
      //bring the hand into the start target
      event_code = E_RETURN_TO_START;
      tickCount = TaskwideParams[K_TIME_TO_START];
      MovOnTraj = 0;
      t_step = 0;
      targetA_state = 1;
      cuetarget_state=CueType+1;
      during:
      //turn on the hand feedback when the hand is in the start target
      handtarget_state = HandInTgtLogical[Trial_Protocol[START_TARGET_COL]];
    state HoldAtStart2/
      handtarget_state = 0;
    state Setup_VP_Trial/
      Vcontrolpt_row[1] = Trial_Protocol[CONTROL_PT0_COL];
      Vcontrolpt_row[2] = Trial_Protocol[CONTROL_PTV1_COL];
      Vcontrolpt_row[3] = Trial_Protocol[CONTROL_PTV2_COL];
      Vcontrolpt_row[4] = Trial_Protocol[CONTROL_PT3_COL];
      Pcontrolpt_row[1] = Trial_Protocol[CONTROL_PT0_COL];
      Pcontrolpt_row[2] = Trial_Protocol[CONTROL_PTP1_COL];
      Pcontrolpt_row[3] = Trial_Protocol[CONTROL_PTP2_COL];
      Pcontrolpt_row[4] = Trial_Protocol[CONTROL_PT3_COL];
      [last_control_ptV] = findLastCtlPt(Vcontrolpt_row[1],Vcontrolpt_row[2],Vcontrolpt_row[3],Vcontrolpt_row[4]);
      [last_control_ptP] = findLastCtlPt(Pcontrolpt_row[1],Pcontrolpt_row[2],Pcontrolpt_row[3],Pcontrolpt_row[4]);
      SegStartPos[1] = CuePos[1];
      SegStartPos[2] = CuePos[2];
      segcount = 1;
      MovOnTraj = 1;
      t_step = 0;
    state Setup_V_Trial/
      Vcontrolpt_row[1] = Trial_Protocol[CONTROL_PT0_COL];
      Vcontrolpt_row[2] = Trial_Protocol[CONTROL_PTV1_COL];
      Vcontrolpt_row[3] = Trial_Protocol[CONTROL_PTV2_COL];
      Vcontrolpt_row[4] = Trial_Protocol[CONTROL_PT3_COL];
      Pcontrolpt_row[1] = Trial_Protocol[CONTROL_PT0_COL];
      Pcontrolpt_row[2] = -1;
      Pcontrolpt_row[3] = -1;
      Pcontrolpt_row[4] = -1;
      [last_control_ptV] = findLastCtlPt(Vcontrolpt_row[1],Vcontrolpt_row[2],Vcontrolpt_row[3],Vcontrolpt_row[4]);
      [last_control_ptP] = findLastCtlPt(Pcontrolpt_row[1],Pcontrolpt_row[2],Pcontrolpt_row[3],Pcontrolpt_row[4]);
      SegStartPos[1] = CuePos[1];
      SegStartPos[2] = CuePos[2];
      segcount = 1;
      MovOnTraj = 1;
      t_step = 0;
    state Setup_P_Trial/
      Vcontrolpt_row[1] = Trial_Protocol[CONTROL_PT0_COL];
      Vcontrolpt_row[2] = -1;
      Vcontrolpt_row[3] = -1;
      Vcontrolpt_row[4] = -1;
      Pcontrolpt_row[1] = Trial_Protocol[CONTROL_PT0_COL];
      Pcontrolpt_row[2] = Trial_Protocol[CONTROL_PTP1_COL];
      Pcontrolpt_row[3] = Trial_Protocol[CONTROL_PTP2_COL];
      Pcontrolpt_row[4] = Trial_Protocol[CONTROL_PT3_COL];
      [last_control_ptV] = findLastCtlPt(Vcontrolpt_row[1],Vcontrolpt_row[2],Vcontrolpt_row[3],Vcontrolpt_row[4]);
      [last_control_ptP] = findLastCtlPt(Pcontrolpt_row[1],Pcontrolpt_row[2],Pcontrolpt_row[3],Pcontrolpt_row[4]);
      SegStartPos[1] = CuePos[1];
      SegStartPos[2] = CuePos[2];
      segcount = 1;
      MovOnTraj = 1;
      t_step = 0;
    state CueEndHoldP/
      //pause at the end of the cue
      event_code = E_HOLD_POS;
      //tickCount = TaskwideParams[K_HOLDTIME];
      MovOnTraj = 1;
      play_tone = 2;
      tickCount = 500;
      //controlpt_row[1] = Trial_Protocol[last_control_pt3];
      //controlpt_row[2] = Trial_Protocol[last_control_pt3];
      //controlpt_row[3] = -1;
      //controlpt_row[4] = -1;
      t_step = 1;
    state ImitationStimCounterP1/
      // The hand is in the start position so start incrementing t_step
      event_code = E_INCREMENTING_TSTEP1;
      //play_tone = 0;
      play_tone = 1;
      targetB_row = Trial_Protocol[REACH_TARGET_COL];
      targetB_state = 0;
      targetV_row = Trial_Protocol[VIS_TARGET_COL];
      handtarget_state = 0; //Trial_Protocol[HAND_VIS_COL];
      t_step = 0;
      during:
      on e_clk: t_step = t_step + (1/ (Trial_Protocol[STIM_DUR_COL]/1000 * 1000)); //increment t_step on each clock cycle
    state CueEndHoldP1/
      //pause at the end of the cue
      tickCount = TaskwideParams[K_HOLDTIME];
      MovOnTraj = 1;
      //play the tone twice to signal the end of the cue period
      play_tone = 1;
      t_step = 1;
    state ReturnToStartP/
      //pause at the end of the cue
      event_code = E_ROBOT_RETURN_TO_START;
      targetV_state = 0; //shut off the cursor on the return
      handtarget_state = 0;
      SegStartPos[1] = 0.0;
      SegStartPos[2] = 0.0;
      segcount = 0;
      Vcontrolpt_row[1] = Trial_Protocol[START_TARGET_COL];
      Vcontrolpt_row[2] = -1;
      Vcontrolpt_row[3] = -1;
      Vcontrolpt_row[4] = -1;
      Pcontrolpt_row[1] = Trial_Protocol[START_TARGET_COL];
      Pcontrolpt_row[2] = -1;
      Pcontrolpt_row[3] = -1;
      Pcontrolpt_row[4] = -1;
      MovOnTraj = 0;
      t_step = 0;
      tickCount = TaskwideParams[K_TIME_TO_START];
      during:
      //on e_clk:  t_step = t_step - (1/ (Trial_Protocol[STIM_DUR_COL]/1000 * 1000));
    state CueGoHoldP/
      //pause at the end of the movement return
      tickCount = ramp_time;
      handtarget_state = 1;
      //release the hand
      enable_controller = 0;
    state HoldInStart1/
      //make sure subjects hand remains in start
      tickCount = 50;
    state GoCue/
      event_code = E_GO_CUE;
      targetA_state = 0;
      targetB_state = 0;
      handtarget_state = 1*HandInTgtLogical[Trial_Protocol[START_TARGET_COL]];
      play_tone = 3;
      tickCount = Trial_Protocol[MAX_MOVE_TIME_COL];
      handmovement = handmovement_init;
      showhandmovement = 0;
      during:
      HandMoving[1] = abs(HandVelocity[1]) >= TaskwideParams[K_HAND_VEL];
      HandMoving[2] = abs(HandVelocity[2]) >= TaskwideParams[K_HAND_VEL];
      %HandMoving[3] = abs(HandVelocity[3]) >= TaskwideParams[K_HAND_VEL];
      %HandMoving[4] = abs(HandVelocity[4]) >= TaskwideParams[K_HAND_VEL];
      //shut off the hand feedback when the hand begins moving
      handtarget_state = 2*HandInTarget[Trial_Protocol[START_TARGET_COL]];
    state MovingState/
      // If movement started, check arm velocity to detect movement offset
      event_code = E_MOVE_ON;
      handtarget_state = handtarget_state*Trial_Protocol[HAND_VIS_COL];
      //if (Trial_Protocol[HAND_VIS_COL]==0)
      //	handtarget_state = 0;
      //end
      during:
      HandMoving[1] = abs(HandVelocity[1]) >= TaskwideParams[K_HAND_VEL];
      HandMoving[2] = abs(HandVelocity[2]) >= TaskwideParams[K_HAND_VEL];
      %HandMoving[3] = abs(HandVelocity[3]) >= TaskwideParams[K_HAND_VEL];
      %HandMoving[4] = abs(HandVelocity[4]) >= TaskwideParams[K_HAND_VEL];
      movVelThreshHit = (HandMoving[1] || HandMoving[2]); %|| HandMoving[3] || HandMoving[4]);
      handmovement[1][stateiter] = HandPos[1];
      handmovement[2][stateiter] = HandPos[2];
      on e_clk: stateiter = stateiter+1;
    state MovementTimeout/
      event_code = E_MOVE_TIMEOUT;
      //handtarget_state = 0;
      //event_code = 50;
    state HandStill/
      // check if the hand velocity is still below threshold
      event_code = E_HOLDING_STILL;
      tickCount = Trial_Protocol[HOLD_TIME_COL];
      during:
      HandMoving[1] = abs(HandVelocity[1]) >= TaskwideParams[K_HAND_VEL];
      HandMoving[2] = abs(HandVelocity[2]) >= TaskwideParams[K_HAND_VEL];
      %HandMoving[3] = abs(HandVelocity[3]) >= TaskwideParams[K_HAND_VEL];
      %HandMoving[4] = abs(HandVelocity[4]) >= TaskwideParams[K_HAND_VEL];
      movVelThreshHit = (HandMoving[1] || HandMoving[2]); %|| HandMoving[3] || HandMoving[4]);
      handmovement[1][stateiter] = HandPos[1];
      handmovement[2][stateiter] = HandPos[2];
      on e_clk: stateiter = stateiter+1;
    state ShowHandFeedback/
      event_code = E_SHOW_FEEDBACK;
      Vcontrolpt_row[1] = Trial_Protocol[CONTROL_PT0_COL];
      Vcontrolpt_row[2] = Trial_Protocol[CONTROL_PTV1_COL];
      Vcontrolpt_row[3] = Trial_Protocol[CONTROL_PTV2_COL];
      Vcontrolpt_row[4] = Trial_Protocol[CONTROL_PT3_COL];
      showhandmovement = 1;
      tickCount = Trial_Protocol[FEEDBACK_TIME_COL];
    state ShowHandFeedback1/
      event_code = E_SHOW_FEEDBACK;
      Vcontrolpt_row[1] = Trial_Protocol[CONTROL_PT0_COL];
      Vcontrolpt_row[2] = Trial_Protocol[CONTROL_PTP1_COL];
      Vcontrolpt_row[3] = Trial_Protocol[CONTROL_PTP2_COL];
      Vcontrolpt_row[4] = Trial_Protocol[CONTROL_PT3_COL];
      showhandmovement = 1;
      HandPos_end[1]=HandPos[1];
      HandPos_end[2]=HandPos[2];
      tickCount = Trial_Protocol[FEEDBACK_TIME_COL];
    state EndOfTrial/
      // Turn off the target, set the post-trial delay
      event_code = E_END_TRIAL;
      targetA_state = 0;
      handtarget_state = 0;
      tickCount = Trial_Protocol[DELAY_POST_TRIAL_COL];
      showhandmovement = 0;
    InitPauseTrial -> EndOfTrial : [taskbtn==4]
    ShowStartTarget -> InitPauseTrial [order 2] : [CueType==4]
        | // analogous with trial type
    ShowStartTarget -> RampOnController [order 1] : [CueType~=4 && after(1,e_clk)]
    RampOnController -> MoveToStart : after(ramp_time, e_clk)
    MoveToStart -> HoldAtStart : [after(tickCount,e_clk) && HandInTarget[Trial_Protocol[START_TARGET_COL]] ]/
        | t_step = 0;
        | //HandInTarget[Trial_Protocol[CONTROL_PT1_COL]] &&
    HoldAtStart -> HoldAtStart2 : after(500,e_clk)/
        | play_tone = 0;
    (junction 197) -> Setup_VP_Trial [order 1] : [CueType >= 2]
    HoldAtStart2 -> (junction 197) : [after((tickCount-500),e_clk)]/
        | t_step = 0;
        | cuetarget_state=0;
        | //play_tone = 1;
        | //HandInTarget[Trial_Protocol[CONTROL_PT1_COL]] &&
    (junction 197) -> Setup_P_Trial [order 3] : [CueType == 1]
    (junction 197) -> Setup_V_Trial [order 2] : [CueType == 0]
    Setup_VP_Trial -> ImitationStimCounterP1 : after(1,e_clk)
    Setup_P_Trial -> ImitationStimCounterP1 : after(1,e_clk)
    Setup_V_Trial -> ImitationStimCounterP1 : after(1,e_clk)
    ImitationStimCounterP1 -> CueEndHoldP : [(t_step >= 1)]/
        | t_step = 1;
        | //SegStartPos[1] = CuePos[1];
        | //SegStartPos[2] = CuePos[2];
        | //&& HandInTarget[Trial_Protocol[last_control_pt]] == 1
        | //if proprioceptively cued, pause
        | //then return hand to start position
    CueEndHoldP -> CueEndHoldP1 : after(tickCount,e_clk)
    CueEndHoldP1 -> ReturnToStartP : after(tickCount,e_clk)
    ReturnToStartP -> CueGoHoldP : after(tickCount,e_clk)
        | //when the hand returns to the start position
    CueGoHoldP -> HoldInStart1 : // is the hand in the target?
        | [HandInTarget[targetA_row] == 1]
    HoldInStart1 -> CueGoHoldP [order 2] : [HandInTarget[targetA_row]==0]
    HoldInStart1 -> GoCue [order 1] : after(tickCount,e_clk)
    GoCue -> MovementTimeout [order 1] : after(tickCount,e_clk)
    GoCue -> MovingState [order 2] : [HandInTarget[targetA_row]==0]/ // || (HandMoving[1] || HandMoving[2] || HandMoving[3] || HandMoving[4])]/
        | //if hand left start position or started moving
        | movVelThreshHit = 0;
        | stateiter = 1;
        | handtarget_state = 0;
    MovingState -> MovementTimeout [order 2] : //check from time first entered the state
        | [(stateiter > Trial_Protocol[MAX_MOVE_TIME_COL])]
    MovementTimeout -> EndOfTrial
    MovingState -> HandStill [order 1] : [stateiter>1000 && !movVelThreshHit && after(1,e_clk)]
    HandStill -> MovingState [order 1] : [movVelThreshHit && after(1,e_clk)]
    HandStill -> ShowHandFeedback [order 2] : [CueType ==0 && after(tickCount,e_clk)]/
        | HandPos_end[1]=HandPos[1];
        | HandPos_end[2]=HandPos[2];
    HandStill -> EndOfTrial [order 3] : [CueType >= 2 && after(tickCount,e_clk)]/
        | HandPos_end[1]=HandPos[1];
        | HandPos_end[2]=HandPos[2];
    HandStill -> ShowHandFeedback1 [order 4] : [CueType ==1 && after(tickCount,e_clk)]/
        | HandPos_end[1]=HandPos[1];
        | HandPos_end[2]=HandPos[2];
    ShowHandFeedback -> (junction 213) : after(tickCount,e_clk)
    ShowHandFeedback1 -> (junction 213) : after(tickCount,e_clk)
    (junction 213) -> EndOfTrial : //e_EndReachBtn/
        | //event_code = 50;
  state Initialize/
    //Initialization state
    targetA_state = 0;
    targetB_state = 0;
    targetV_state = 0;
    targetP_state = 0;
    handtarget_state = 1;
    handtarget_row = 3;
    Repeat_Trial_Flag = 0;
    ramp_time = TaskwideParams[K_ROBOT_RAMP_TIME];
    enable_controller = 0;
    segcount = -1
    handtarget_row = TaskwideParams[K_HAND_TARGET];
    handtarget_state = 1;
  state Inter_Trial_State/
    // Turn off target, reset the event code, and send the
    //e_Trial_End Stateflow event to indicate that the trial is over.
    event_code = 0;
    targetA_state = 0;
    targetB_state = 0;
    handtarget_state = 1;
    Repeat_Trial_Flag = 0;
    segcount = -1;
    e_Trial_End;
    HandPos_end[1]=0;
    HandPos_end[2]=0;
    handtarget_state = 0;
  state RobotRampDown/
    enable_controller = 0;
  note: ?
  (default) -> Initialize
  Initialize -> ShowStartTarget
  Inter_Trial_State -> ShowStartTarget : // has a a specified period of
      | // time occured?
      | after(tickCount, e_clk)
  (junction 116) -> Inter_Trial_State [order 1] : [enable_controller == 0]
  MainTrial -> (junction 116) : e_ExitTrialNow/
      | tickCount = 1;
      | // e_ExitTrialNow event occurs if the
      | // Dex pause is pressed by the operator
  (junction 116) -> RobotRampDown [order 2] : [enable_controller == 1]
  EndOfTrial -> Inter_Trial_State : after(tickCount,e_clk)
  RobotRampDown -> Inter_Trial_State : after(ramp_time,e_clk)
  data: cp1 function_input double; cp2 function_input double; cp3 function_input double; cp4 function_input double; lcp function_output double; t function_output double; HandMoving output boolean size=4; event_code output uint16 [0..] =0; targetA_row output [1..32]; targetA_state output double; targetB_row output double; targetB_state output double; tickCount local double; Trial_Protocol input double; HandInTarget input double; HandInTgtLogical input double; TaskwideParams input double; HandPos input double size=2; HandVelocity input double; targetV_row output double; targetV_state output double; t_step output double; Vcontrolpt_row output double size=4; Pcontrolpt_row output double size=4; SegStartPos output double size=2; segcount output double; handtarget_row output double; handtarget_state output double; movVelThreshHit local boolean; CueType output double; ramp_time local double; enable_controller output boolean; targetP_state output double; MovOnTraj output double; handmovement output double size=[2 8000] =0; showhandmovement output double; stateiter output double; play_tone output double; Repeat_Trial_Flag output double; last_control_ptV local double =0; last_control_ptP local double =0; CuePos input double size=2; handmovement_init local double size=[2 8000]; targetC_row output double; HandPos_end output double size=2; cuetarget_state output double; cuetarget_row output double; taskbtn input double
  data targetA_row settings: description=index of the row currently being used in the TargetTable
  events: e_clk input RISING_EDGE_EVENT; e_ExitTrialNow input EITHER_EDGE_EVENT; e_Trial_End output EITHER_EDGE_EVENT
  function [lcp,t]  = findLastCtlPt(cp1,cp2,cp3,cp4):
    | function [lcp,t]  = findLastCtlPt(cp1,cp2,cp3,cp4)
    | 
    | %find the index to the last control point in the TP table
    | 
    | 
    | lcp = 0;
    | indlcp = 0;
    | 
    | if (cp4 > 0)
    | 	lcp = cp4;
    |     indlcp = 4;
    |     t = 0;
    | elseif (cp3 > 0)
    | 	lcp = cp3;
    |     indlcp = 3;
    |     t = 0;
    | elseif (cp2 > 0)
    | 	lcp = cp2;
    |     indlcp = 2;
    |     t = 0;
    | else
    | 	lcp = cp1;
    |     indlcp = 1;
    |     t = 1;
    | end
